simulink model "Receiver"  (R2024b)
settings: Solver=VariableStepAuto  StartTime=0.0  StopTime=inf  RelTol=1e-3
libraries: dspfdesign x6, dspsigops x2, simulink x1, sdrrlib x1
settings Model: Creator=Ben Paxson  LastModifiedBy=Ben Paxson
settings DebuggingCC: UnderSpecifiedDimensionMsg=warning

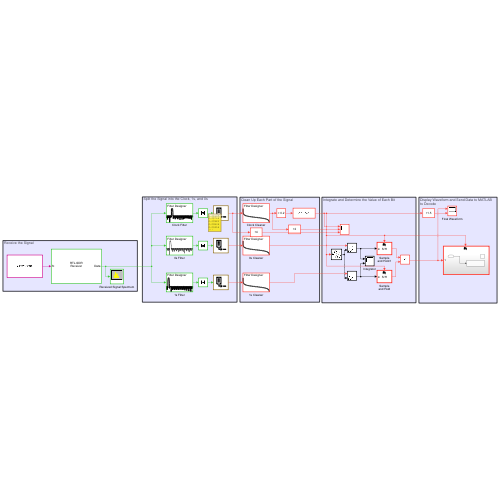
[thumbnail: Simulink's stored preview of the top-level diagram]
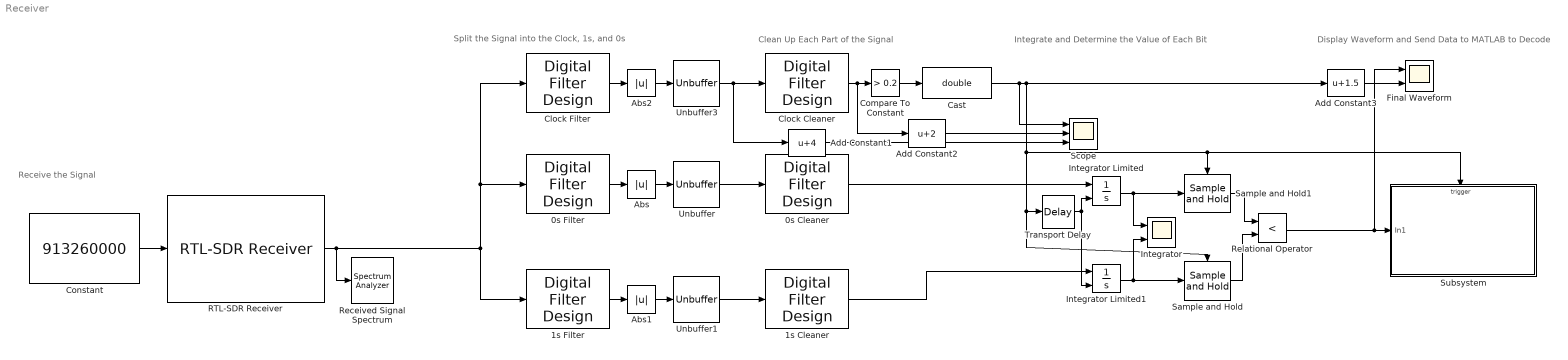
== system Receiver ==
  note: Display Waveform and Send Data to MATLAB
      | to Decode
  note: Integrate and Determine the Value of Each Bit
  note: Clean Up Each Part of the Signal
  note: Split the Signal into the Clock, 1s, and 0s
  note: Receive the Signal
  0s Cleaner : dspfdesign/Digital Filter Design  mwdsp_browser_bugfix_var=off
  0s Filter : dspfdesign/Digital Filter Design  mwdsp_browser_bugfix_var=off
  1s Cleaner : dspfdesign/Digital Filter Design  mwdsp_browser_bugfix_var=off
  1s Filter : dspfdesign/Digital Filter Design  mwdsp_browser_bugfix_var=off
  Abs : Abs  SaturateOnIntegerOverflow=off
  Abs1 : Abs  SaturateOnIntegerOverflow=off
  Abs2 : Abs  SaturateOnIntegerOverflow=off
  Add Constant1 : Bias  Bias=4  SaturateOnIntegerOverflow=off
  Add Constant2 : Bias  Bias=2  SaturateOnIntegerOverflow=off
  Add Constant3 : Bias  Bias=1.5  SaturateOnIntegerOverflow=off
  Cast : DataTypeConversion  OutDataTypeStr=double  SaturateOnIntegerOverflow=off  RndMeth=Floor
  Clock Cleaner : dspfdesign/Digital Filter Design  mwdsp_browser_bugfix_var=off
  Clock Filter : dspfdesign/Digital Filter Design  mwdsp_browser_bugfix_var=off
  Compare To Constant : simulink/Logic and Bit Operations/Compare To Constant  relop=>  const=0.2  OutDataTypeStr=uint8
  Constant : Constant  Value=913260000
  Final Waveform : Scope  NumInputPorts=2
  Integrator : Scope  NumInputPorts=2
  Integrator Limited : Integrator  ExternalReset=either  UpperSaturationLimit=1  LowerSaturationLimit=0
  Integrator Limited1 : Integrator  ExternalReset=either  UpperSaturationLimit=1  LowerSaturationLimit=0
  RTL-SDR Receiver : sdrrlib/RTL-SDR Receiver  IPAddress=0  CenterFrequencySource=Input port  CenterFrequency=102.5e6  GainSource=AGC  Gain=0  ADCRate=300000  FrequencyCorrection=53  LostSamplesOutputPort=off  LatencyOutputPort=off  OutputDataType=double  FrameLength=1024  EnableBurstMode=off  NumFramesInBurst=20  sobjType=sdrr.internal.SDRRTLReceiverSL  dataUDPPort=-1  ctrlUDPPort=-1  subDeviceList=nosubdev  sdrBlockType=SDRBlockTypeSLT.SDRRxBlock  requester=UNUSED_BY_SFCN  sdrExecutionMode=SDRExecutionModeSLT.ExecModeHW  BypassUserLogic=off  DecimatorSelect=DDC decimator  SourceSelect=RF data  SineAmplitude=16000  EnableInternalClock=off  BypassIQBalance=off  IFBandwidth=40e6  ADCRateSource=Dialog  IntermediateFrequency=0  DecimationFactorSource=Dialog  DecimationFactor=512  RFFrequencyIsTunable=logical(1)  SampleTime=(1024)/(300000)  IFBandwidthSource=Dialog  SineFrequency=30000  BypassDCBlockingFilter=off  IntermediateFrequencySource=Dialog  IQBalanceCoefficients=64  SkipAllHardwareResetAndInitialization=off  EnableIQCalibrationTable=on  CacheIQCalibrationTable=off  EnableOffsetTuning=off  EnableRTLAGC=off  EnableTestMode=off  EnableTunerAGC=on  FrequencyCorrectionSource=Dialog  NumMLBuffers=128  NumUSBBuffers=16  RTLCrystalFrequency=28800000  TunerCrystalFrequency=28800000
  Received Signal Spectrum : SpectrumAnalyzer  WindowPosition=[8.000000,40.000000,1520.000000,784.000000,]  ScopeFrameLocation=window  WindowInvariantSamplesPerUpdate=on  Span=300000  StartFrequency=-150000  StopFrequency=150000  YLimits=[-44.63934948,14.13153474]
  Relational Operator : RelationalOperator  Operator=<  OutDataTypeStr=boolean  RndMeth=Simplest  InputSameDT=off
  Sample and Hold : dspsigops/Sample and Hold  trig=Either edge  initCond=0  latchinput=off
  Sample and Hold1 : dspsigops/Sample and Hold  trig=Either edge  initCond=0  latchinput=off
  Scope : Scope  NumInputPorts=3
  Subsystem : Subsystem
  Transport Delay : TransportDelay  DelayTime=1e-6
  Unbuffer : Unbuffer
  Unbuffer1 : Unbuffer
  Unbuffer3 : Unbuffer
  wires:
  RTL-SDR Receiver/1 -> Clock Filter/1, 0s Filter/1, 1s Filter/1, Received Signal Spectrum/1
  Constant/1 -> RTL-SDR Receiver/1
  0s Filter/1 -> Abs/1
  1s Filter/1 -> Abs1/1
  Unbuffer/1 -> 0s Cleaner/1
  Abs1/1 -> Unbuffer1/1
  Abs/1 -> Unbuffer/1
  Unbuffer3/1 -> Add Constant1/1, Clock Cleaner/1
  Abs2/1 -> Unbuffer3/1
  Clock Filter/1 -> Abs2/1
  Integrator Limited/1 -> Integrator/1, Sample and Hold1/1
  Sample and Hold1/1 -> Relational Operator/1
  Sample and Hold/1 -> Relational Operator/2
  Transport Delay/1 -> Integrator Limited1/2, Integrator Limited/2
  Integrator Limited1/1 -> Sample and Hold/1, Integrator/2
  Clock Cleaner/1 -> Add Constant2/1, Compare To Constant/1
  Compare To Constant/1 -> Cast/1
  Cast/1 -> Scope/1, Add Constant3/1, Subsystem/Trigger, Sample and Hold1/Trigger, Transport Delay/1, Sample and Hold/Trigger
  Unbuffer1/1 -> 1s Cleaner/1
  Add Constant3/1 -> Final Waveform/2
  Relational Operator/1 -> Subsystem/1(In1), Final Waveform/1
  1s Cleaner/1 -> Integrator Limited1/1
  Add Constant1/1 -> Scope/3
  Add Constant2/1 -> Scope/2
  0s Cleaner/1 -> Integrator Limited/1

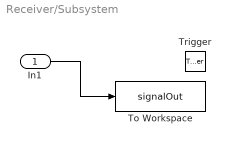
== system Receiver/Subsystem ==
  In1 : Inport
  Trigger : TriggerPort  TriggerType=either  VariantControl=(inherit)  PortDimensions=1
  To Workspace : ToWorkspace  VariableName=signalOut  SampleTime=-1
  wires:
  In1/1 -> To Workspace/1
